simulink model "Task4_Robust_MRAC"  (R2024b)
settings: Solver=ode45  StartTime=0.0  StopTime=120  MaxStep=0.02  RelTol=1e-7  AbsTol=1e-9
settings Model: Creator=LAPTOPASADI  LastModifiedBy=LAPTOPASADI
settings DataIOCC: SaveOutput=off  SignalLogging=off  SaveTime=off  ReturnWorkspaceOutputs=off

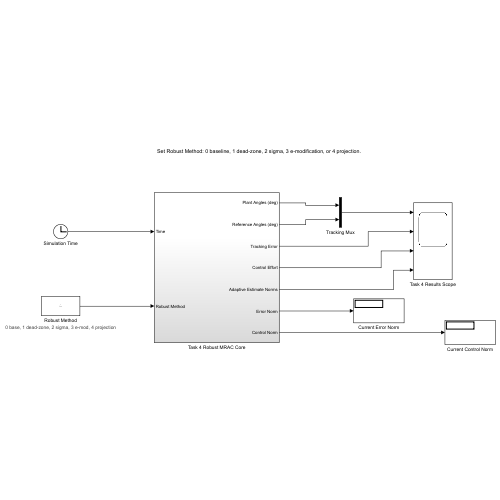
[thumbnail: Simulink's stored preview of the top-level diagram]
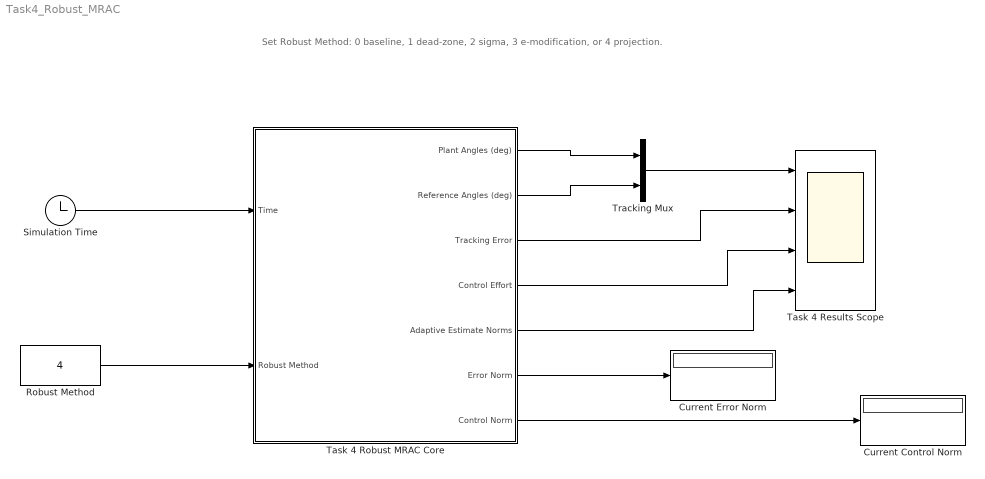
== system Task4_Robust_MRAC ==
  note: Set Robust Method: 0 baseline, 1 dead-zone, 2 sigma, 3 e-modification, or 4 projection.
  Current Control Norm : Display
  Current Error Norm : Display
  Robust Method : Constant  Value=4
      settings: AttributesFormatString=0 base, 1 dead-zone, 2 sigma, 3 e-mod, 4 projection
  Simulation Time : Clock
  Task 4 Results Scope : Scope  NumInputPorts=4
  Task 4 Robust MRAC Core : Subsystem
  Tracking Mux : Mux  Inputs=2
  wires:
  Simulation Time/1 -> Task 4 Robust MRAC Core/1(Time)
  Robust Method/1 -> Task 4 Robust MRAC Core/2(Robust Method)
  Task 4 Robust MRAC Core/1(Plant Angles (deg)) -> Tracking Mux/1
  Task 4 Robust MRAC Core/2(Reference Angles (deg)) -> Tracking Mux/2
  Tracking Mux/1 -> Task 4 Results Scope/1
  Task 4 Robust MRAC Core/3(Tracking Error) -> Task 4 Results Scope/2
  Task 4 Robust MRAC Core/4(Control Effort) -> Task 4 Results Scope/3
  Task 4 Robust MRAC Core/5(Adaptive Estimate Norms) -> Task 4 Results Scope/4
  Task 4 Robust MRAC Core/6(Error Norm) -> Current Error Norm/1
  Task 4 Robust MRAC Core/7(Control Norm) -> Current Control Norm/1

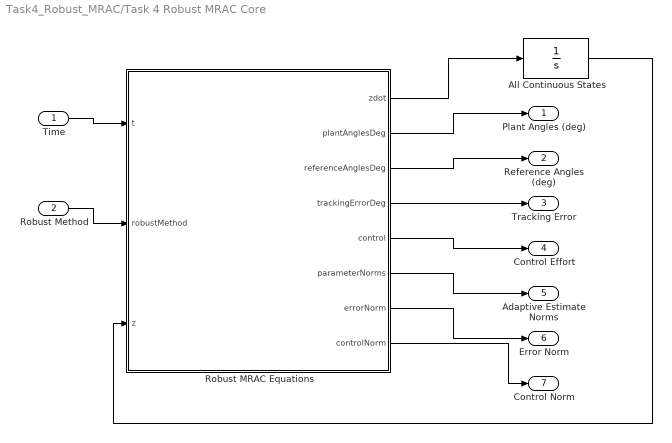
== system Task4_Robust_MRAC/Task 4 Robust MRAC Core ==
  Time : Inport
  Robust Method : Inport  Port=2
  All Continuous States : Integrator  InitialCondition=[0;0;0;0;0;0;0;0;0;0;0;0;0;-0.66823529411764704;0;0;-0.66823529411764704;0;-0.093784508916032808;0;-0.084095775670305087;-0.093784508916032808;0;-0.084095775670305087;-0.020546127010358625;0;0.38386217602841338;-0.020546127010358625;0;0.38386217602841338;0;0.66823529411764704;0;0.093784508916032808;0;0.084095775670305087;0.020546127010358625;0;-0.38386217602841338;0;0.15647058823529411;0;0;-0.0016705882352941175;0;-0.018538798274099509;0;-0.011825968453636653;-0.00023446127229008202;0;-0.00021023943917576274;-0.0040614437113499612;0;0.053980618503995631;-5.1365317525896568e-05;0;0.00095965544007103345]
  Robust MRAC Equations : MATLAB Function  TreatAsAtomicUnit=on
  Plant Angles (deg) : Outport
  Reference Angles (deg) : Outport  Port=2
  Tracking Error : Outport  Port=3
  Control Effort : Outport  Port=4
  Adaptive Estimate Norms : Outport  Port=5
  Error Norm : Outport  Port=6
  Control Norm : Outport  Port=7
  wires:
  Time/1 -> Robust MRAC Equations/1(t)
  Robust Method/1 -> Robust MRAC Equations/2(robustMethod)
  All Continuous States/1 -> Robust MRAC Equations/3(z)
  Robust MRAC Equations/1(zdot) -> All Continuous States/1
  Robust MRAC Equations/2(plantAnglesDeg) -> Plant Angles (deg)/1
  Robust MRAC Equations/3(referenceAnglesDeg) -> Reference Angles (deg)/1
  Robust MRAC Equations/4(trackingErrorDeg) -> Tracking Error/1
  Robust MRAC Equations/5(control) -> Control Effort/1
  Robust MRAC Equations/6(parameterNorms) -> Adaptive Estimate Norms/1
  Robust MRAC Equations/7(errorNorm) -> Error Norm/1
  Robust MRAC Equations/8(controlNorm) -> Control Norm/1

== matlab function Task4_Robust_MRAC/Task 4 Robust MRAC Core/Robust MRAC Equations ==
  data: t input; zdot output; robustMethod input; z input; plantAnglesDeg output; referenceAnglesDeg output; trackingErrorDeg output; control output; parameterNorms output; errorNorm output; controlNorm output
function [zdot,plantAnglesDeg,referenceAnglesDeg,trackingErrorDeg,control,parameterNorms,errorNorm,controlNorm] = robustMRAC(t,robustMethod,z)
%#codegen
% Standalone Task 4 equations with one selector for all robust laws.

x = z(1:6);
xm = z(7:12);
KxHat = reshape(z(13:30),6,3);
KrHat = reshape(z(31:39),3,3);
ThetaHat = reshape(z(40:57),6,3);
KxStar = [0 -0.093784508916032808 -0.020546127010358625;-0.66823529411764704 0 0;0 -0.084095775670305087 0.38386217602841338;0 -0.093784508916032808 -0.020546127010358625;-0.66823529411764704 0 0;0 -0.084095775670305087 0.38386217602841338];
KrStar = [0 0.093784508916032808 0.020546127010358625;0.66823529411764704 0 0;0 0.084095775670305087 -0.38386217602841338];
ThetaStar = [0 -0.018538798274099509 -0.0040614437113499612;0.15647058823529411 0 0;0 -0.011825968453636653 0.053980618503995631;0 -0.00023446127229008202 -5.1365317525896568e-05;-0.0016705882352941175 0 0;0 -0.00021023943917576274 0.00095965544007103345];

reference = zeros(3,1);
if t >= 1
    tau = t-1;
    weights = [0.30,0.24,0.19,0.15,0.12];
    peaks = (pi/180)*[10;10;15];
    amplitude = peaks*weights;
    frequency = [0.31,0.53,0.79,1.07,1.37; ...
                 0.37,0.61,0.89,1.19,1.43; ...
                 0.43,0.67,0.97,1.27,1.51];
    reference = sum(amplitude.*sin(frequency*tau),2);
end

dOverB = 1.2e-6/3.13e-5;
G = [0,0.175/0.0043,dOverB/0.0043; ...
     0.085/0.0142,0,0; ...
     0,dOverB/0.0176,-0.175/0.0176];
aP = (0.0142-0.0176)/0.0043;
aQ = (0.0176-0.0043)/0.0142;
aR = (0.0043-0.0142)/0.0176;
Htrue = [aP,0,0,-0.01,0,0; ...
         0,aQ,0,0,-0.01,0; ...
         0,0,aR,0,0,-0.01];
B = [zeros(3,3);G];

p = x(4);
q = x(5);
rBody = x(6);
Phi = [q*rBody;p*rBody;p*q;p;q;rBody];
control = KxHat.'*x + KrHat.'*reference - ThetaHat.'*Phi;

disturbanceAmplitude = [ ...
    3.0e-4,2.0e-4,1.0e-4; ...
    2.5e-4,2.0e-4,1.5e-4; ...
    2.8e-4,1.8e-4,1.2e-4; ...
    3.0e-3,2.0e-3,1.0e-3; ...
    2.8e-3,1.8e-3,1.2e-3; ...
    3.2e-3,2.1e-3,1.1e-3];
disturbanceFrequency = [ ...
    0.17,0.43,0.79;0.23,0.53,0.91;0.29,0.61,1.03; ...
    0.19,0.47,0.83;0.31,0.67,1.09;0.37,0.73,1.19];
disturbancePhase = [ ...
    0.0,0.4,0.8;0.2,0.6,1.0;0.4,0.8,1.2; ...
    0.6,1.0,1.4;0.8,1.2,1.6;1.0,1.4,1.8];
eta = sum(disturbanceAmplitude.*sin(disturbanceFrequency*t+disturbancePhase),2);
xdot = [x(4:6);G*control+Htrue*Phi]+eta;
xmdot = [xm(4:6);-4*xm(1:3)-4*xm(4:6)+4*reference];

error = x-xm;
P = [1.125*eye(3),0.125*eye(3); ...
     0.125*eye(3),0.15625*eye(3)];
signal = error.'*P*B;
rawKxDot = -50*x*signal;
rawKrDot = -50*reference*signal;
rawThetaDot = 50*Phi*signal;

if robustMethod < 0.5
    KxHatDot = rawKxDot;
    KrHatDot = rawKrDot;
    ThetaHatDot = rawThetaDot;
elseif robustMethod < 1.5
    if sqrt(sum(error.^2)) > 0.026521635489078873
        KxHatDot = rawKxDot;
        KrHatDot = rawKrDot;
        ThetaHatDot = rawThetaDot;
    else
        KxHatDot = zeros(6,3);
        KrHatDot = zeros(3,3);
        ThetaHatDot = zeros(6,3);
    end
elseif robustMethod < 2.5
    sigma = 2.0e-5;
    KxHatDot = rawKxDot-sigma*50*KxHat;
    KrHatDot = rawKrDot-sigma*50*KrHat;
    ThetaHatDot = rawThetaDot-sigma*50*ThetaHat;
elseif robustMethod < 3.5
    leakage = 5.0e-3*sqrt(sum(error.^2));
    KxHatDot = rawKxDot-leakage*50*KxHat;
    KrHatDot = rawKrDot-leakage*50*KrHat;
    ThetaHatDot = rawThetaDot-leakage*50*ThetaHat;
else
    KxHatDot = projectBox(KxHat,rawKxDot,abs(KxStar)+0.002);
    KrHatDot = projectBox(KrHat,rawKrDot,abs(KrStar)+0.002);
    ThetaHatDot = projectBox(ThetaHat,rawThetaDot,abs(ThetaStar)+0.001);
end

zdot = [xdot;xmdot;KxHatDot(:);KrHatDot(:);ThetaHatDot(:)];
plantAnglesDeg = (180/pi)*x(1:3);
referenceAnglesDeg = (180/pi)*xm(1:3);
trackingErrorDeg = (180/pi)*error;
estimateNorm = sqrt(sum(KxHat(:).^2)+sum(KrHat(:).^2)+sum(ThetaHat(:).^2));
parameterError = sqrt(sum((KxHat(:)-KxStar(:)).^2)+ ...
    sum((KrHat(:)-KrStar(:)).^2)+sum((ThetaHat(:)-ThetaStar(:)).^2));
parameterNorms = [estimateNorm;parameterError];
errorNorm = sqrt(sum(error.^2));
controlNorm = sqrt(sum(control.^2));
end

function derivative = projectBox(estimate,proposed,limit)
derivative = proposed;
for k = 1:numel(estimate)
    if estimate(k) > limit(k)
        derivative(k) = min(proposed(k),-100*(estimate(k)-limit(k)));
    elseif estimate(k) < -limit(k)
        derivative(k) = max(proposed(k),100*(-limit(k)-estimate(k)));
    elseif estimate(k) >= limit(k)-1e-12 && proposed(k) > 0
        derivative(k) = 0;
    elseif estimate(k) <= -limit(k)+1e-12 && proposed(k) < 0
        derivative(k) = 0;
    end
end
end
